simulink model "tank_FP"  (R2021b)
settings: Solver=VariableStepAuto  StartTime=0.0  StopTime=30  RelTol=1e-4
undefined symbols (not defined in the file): A, Ak, B, Be, beta, Bh, Bs, C, d, Dh, Discrete, Dm, Ds, Fc, Flp, Hd, Hm_init, Hs_init, Jh, Ke, Kh, Ks, Mm, Ms, noise, Ph, R, Time, tlcAlpha, Ts, xe
libraries: simulink x3, ctrlSharedLib x2, cstblocks x1
settings Model: Creator=buse  LastModifiedBy=buse

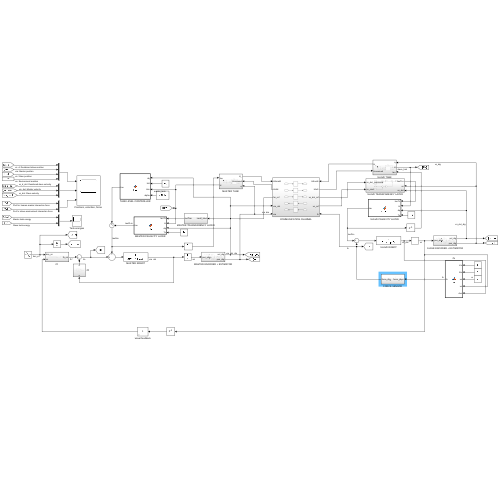
[thumbnail: Simulink's stored preview of the top-level diagram]
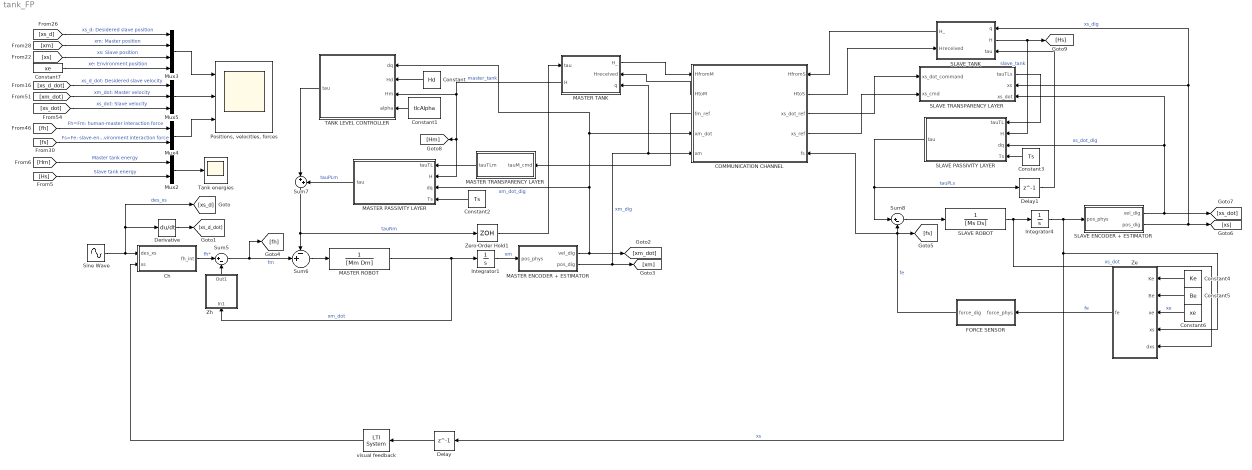
== system tank_FP ==
  COMMUNICATION CHANNEL : Subsystem
      settings: PortSchema="{\"entries\":[{\"content\":{\"sides\":[{\"content\":{\"connectorIds\":[\"In1\",\"Out3\",\"Out4\",\"Out5\",\"In2\"]},\"type\":\"ConnectorPlacement.EquallySpacedRectSide\",\"uuid\":\"1c070cf8-9aa7-4f7b-8e2f-2632c2893f69\"},{\"content\":{\"connectorIds\":[\"In3\",\"Out1\",\"Out2\",\"In4\",\"In5\"],\"side\":\"RIGHT\"},\"type\":\"ConnectorPlacement.EquallySpacedRectSide\",\"uuid\":\"32173565-3523-4dfc-9820-763c87098354\"},{\"content\":{\"connectorIds\":[],\"side\":\"TOP\"},\"type\":\"ConnectorPlacement.EquallySpacedRectSide\",\"uuid\":\"13187df6-bf6f-436e-a2ee-34150977e6a8\"},{\"content\":{\"connectorIds\":[],\"side\":\"HIDDEN\"},\"type\":\"ConnectorPlacement.EquallySpacedRectSide\",\"uuid\":\"1e5bcdd7-6028-40f7-b524-727817e519ff\"}]},\"type\":\"ConnectorPlacement.EquallySpacedConnector\",\"uuid\":\"c84d0440-83b9-4b92-a10a-1f72bb115b54\"}],\"packageUris\":[\"http://schema.mathworks.com/mf0/Connector/R2020b\"],\"version\":\"1.0\"}"
  Ch : Subsystem
  Constant : Constant  Value=Hd
  Constant1 : Constant  Value=tlcAlpha
  Constant2 : Constant  Value=Ts
  Constant3 : Constant  Value=Ts
  Constant4 : Constant  Value=Ke
  Constant5 : Constant  Value=Be
  Constant6 : Constant  Value=xe
  Constant7 : Constant  Value=xe
  Delay : Delay  DelayLength=1  SampleTime=Ts
  Delay1 : Delay  DelayLength=1  SampleTime=Ts
  Derivative : Derivative
  "FORCE SENSOR " : Subsystem
  Integrator1 : Integrator
  Integrator4 : Integrator
  MASTER ENCODER + ESTIMATOR : Subsystem
  MASTER PASSIVITY LAYER : MATLAB Function  TreatAsAtomicUnit=on
  MASTER ROBOT : TransferFcn  Denominator=[Mm Dm]
  MASTER TANK : Subsystem
      settings: PortSchema="{\"entries\":[{\"content\":{\"sides\":[{\"content\":{\"connectorIds\":[\"Out2\",\"In1\",\"In2\"]},\"type\":\"ConnectorPlacement.EquallySpacedRectSide\",\"uuid\":\"482b0a11-f044-49fa-a74d-4dac8b5b787b\"},{\"content\":{\"connectorIds\":[\"In3\",\"Out1\"],\"side\":\"RIGHT\"},\"type\":\"ConnectorPlacement.EquallySpacedRectSide\",\"uuid\":\"b0c369ed-ae40-43d8-b393-bca9f7720d62\"},{\"content\":{\"connectorIds\":[],\"side\":\"TOP\"},\"type\":\"ConnectorPlacement.EquallySpacedRectSide\",\"uuid\":\"ff021616-d6aa-4c0a-874b-a9ebe947c92c\"},{\"content\":{\"connectorIds\":[],\"side\":\"BOTTOM\"},\"type\":\"ConnectorPlacement.EquallySpacedRectSide\",\"uuid\":\"4e18ee96-bca7-41b6-9abb-5b593b41c296\"},{\"content\":{\"connectorIds\":[],\"side\":\"HIDDEN\"},\"type\":\"ConnectorPlacement.EquallySpacedRectSide\",\"uuid\":\"be815b34-35c7-4c6f-8c8b-4a812b3d12e9\"}]},\"type\":\"ConnectorPlacement.EquallySpacedConnector\",\"uuid\":\"78552b8a-5f1c-4815-a807-de98f58b7f2e\"}],\"packageUris\":[\"http://schema.mathworks.com/mf0/Connector/R2020b\"],\"version\":\"1.0\"}"
  MASTER TRANSPARENCY LAYER : Subsystem
  Mux2 : Mux  Inputs=2
  Mux3 : Mux
  Mux4 : Mux  Inputs=2
  Mux5 : Mux  Inputs=3
  "Positions, velocities, forces" : Scope  NumInputPorts=3
  SLAVE ENCODER + ESTIMATOR : Subsystem
  SLAVE PASSIVITY LAYER : MATLAB Function  TreatAsAtomicUnit=on
  SLAVE ROBOT : TransferFcn  Denominator=[Ms Ds]
  SLAVE TANK : Subsystem
      settings: PortSchema="{\"entries\":[{\"content\":{\"sides\":[{\"content\":{\"connectorIds\":[\"In1\",\"Out2\",\"In2\"]},\"type\":\"ConnectorPlacement.EquallySpacedRectSide\",\"uuid\":\"482b0a11-f044-49fa-a74d-4dac8b5b787b\"},{\"content\":{\"connectorIds\":[\"Out1\",\"In3\"],\"side\":\"RIGHT\"},\"type\":\"ConnectorPlacement.EquallySpacedRectSide\",\"uuid\":\"b0c369ed-ae40-43d8-b393-bca9f7720d62\"},{\"content\":{\"connectorIds\":[],\"side\":\"TOP\"},\"type\":\"ConnectorPlacement.EquallySpacedRectSide\",\"uuid\":\"ff021616-d6aa-4c0a-874b-a9ebe947c92c\"},{\"content\":{\"connectorIds\":[],\"side\":\"BOTTOM\"},\"type\":\"ConnectorPlacement.EquallySpacedRectSide\",\"uuid\":\"4e18ee96-bca7-41b6-9abb-5b593b41c296\"},{\"content\":{\"connectorIds\":[],\"side\":\"HIDDEN\"},\"type\":\"ConnectorPlacement.EquallySpacedRectSide\",\"uuid\":\"be815b34-35c7-4c6f-8c8b-4a812b3d12e9\"}]},\"type\":\"ConnectorPlacement.EquallySpacedConnector\",\"uuid\":\"78552b8a-5f1c-4815-a807-de98f58b7f2e\"}],\"packageUris\":[\"http://schema.mathworks.com/mf0/Connector/R2020b\"],\"version\":\"1.0\"}"
  SLAVE TRANSPARENCY LAYER : Subsystem
      settings: PortSchema="{\"entries\":[{\"content\":{\"sides\":[{\"content\":{\"connectorIds\":[\"In1\",\"In2\"]},\"type\":\"ConnectorPlacement.EquallySpacedRectSide\",\"uuid\":\"c8f256d1-8287-4bc6-9264-40c0684f6acd\"},{\"content\":{\"connectorIds\":[\"Out1\",\"In3\",\"In4\"],\"side\":\"RIGHT\"},\"type\":\"ConnectorPlacement.EquallySpacedRectSide\",\"uuid\":\"cb9f571e-93fc-426e-a4f2-aa96ae3bd6b3\"},{\"content\":{\"connectorIds\":[],\"side\":\"TOP\"},\"type\":\"ConnectorPlacement.EquallySpacedRectSide\",\"uuid\":\"b9b91304-f20e-4a66-aa64-b99c686ee85a\"},{\"content\":{\"connectorIds\":[],\"side\":\"HIDDEN\"},\"type\":\"ConnectorPlacement.EquallySpacedRectSide\",\"uuid\":\"c3abcf5a-e3b9-4b9a-a4b1-68c5725be1f4\"}]},\"type\":\"ConnectorPlacement.EquallySpacedConnector\",\"uuid\":\"83907002-acbd-4948-aeba-a43201e13c19\"}],\"packageUris\":[\"http://schema.mathworks.com/mf0/Connector/R2020b\"],\"version\":\"1.0\"}"
  Sine Wave : Sin  Amplitude=A  Frequency=Fc  SampleTime=0
  Sum5 : Sum  Inputs=|+-
  Sum6 : Sum  Inputs=-+|
  Sum7 : Sum  Inputs=|++
  Sum8 : Sum  Inputs=|+-
  TANK LEVEL CONTROLLER : MATLAB Function  TreatAsAtomicUnit=on
  Tank energies : Scope
  Ze : MATLAB Function  TreatAsAtomicUnit=on
  Zero-Order Hold1 : ZeroOrderHold  SampleTime=Ts
  Zh : Subsystem
  visual feedback : cstblocks/LTI System  sys=1  IC=[]
  wires:
  [xs_dot] -> Mux5/3  "xs_dot: Slave velocity"
  Mux5/1 -> "Positions, velocities, forces"/2
  [xs] -> Mux3/3  "xs: Slave position"
  [fh] -> Mux4/1  "Fh=Fm: human-master interaction force"
  Mux4/1 -> "Positions, velocities, forces"/3
  [xm_dot] -> Mux5/2  "xm_dot: Master velocity"
  [xs_d_dot] -> Mux5/1  "xs_d_dot: Desidered slave velocity"
  [xm] -> Mux3/2  "xm: Master position"
  Mux3/1 -> "Positions, velocities, forces"/1
  [fs] -> Mux4/2  "Fs=Fe: slave-environment interaction force"
  Constant7/1 -> Mux3/4  "xe: Environment position"
  [xs_d] -> Mux3/1  "xs_d: Desidered slave position"
  SLAVE ENCODER + ESTIMATOR/2(pos_dig) -> SLAVE TANK/1(q), SLAVE TRANSPARENCY LAYER/3(xs), [xs]  "xs_dig"
  Ze/1(fe) -> "FORCE SENSOR "/1(force_phys)  "fe"
  Constant3/1 -> SLAVE PASSIVITY LAYER/4(Ts)
  Constant6/1 -> Ze/3(xe)  "xe"
  COMMUNICATION CHANNEL/1(HtoM) -> MASTER TANK/1(Hreceived)
  visual feedback/1 -> Ch/2(xs)
  Sum6/1 -> MASTER ROBOT/1
  MASTER PASSIVITY LAYER/1(tau) -> Sum7/2  "tauPLm"
  MASTER TANK/1(H) -> [Hm], MASTER PASSIVITY LAYER/2(H), TANK LEVEL CONTROLLER/3(Hm)  "master_tank"
  MASTER ENCODER + ESTIMATOR/1(vel_dig) -> [xm_dot], TANK LEVEL CONTROLLER/1(dq), COMMUNICATION CHANNEL/4(xm_dot), MASTER PASSIVITY LAYER/3(dq)  "xm_dot_dig"
  MASTER ROBOT/1 -> Zh/1(In1), Integrator1/1  "xm_dot"
  Delay/1 -> visual feedback/1
  MASTER TRANSPARENCY LAYER/1(tauTLm) -> MASTER PASSIVITY LAYER/1(tauTL)
  COMMUNICATION CHANNEL/4(xs_dot_ref) -> SLAVE TRANSPARENCY LAYER/1(xs_dot_command)
  Sum7/1 -> Zero-Order Hold1/1, Sum6/1  "tauRm"
  Integrator1/1 -> MASTER ENCODER + ESTIMATOR/1(pos_phys)  "xm"
  Constant4/1 -> Ze/1(Ke)
  SLAVE ENCODER + ESTIMATOR/1(vel_dig) -> [xs_dot], SLAVE TRANSPARENCY LAYER/4(xs_dot), SLAVE PASSIVITY LAYER/3(dq)  "xs_dot_dig"
  Sum5/1 -> Sum6/2, [fh]  "fm"
  Constant1/1 -> TANK LEVEL CONTROLLER/4(alpha)
  Sine Wave/1 -> Ch/1(des_xs), Derivative/1, [xs_d]  "des_xs"
  Sum8/1 -> SLAVE ROBOT/1
  Zh/1(Out1) -> Sum5/2
  SLAVE TANK/2(H) -> [Hs], SLAVE PASSIVITY LAYER/2(H)  "slave_tank"
  Constant5/1 -> Ze/2(Be)
  COMMUNICATION CHANNEL/2(fm_ref) -> MASTER TRANSPARENCY LAYER/1(tauM_cmd)
  SLAVE PASSIVITY LAYER/1(tau) -> Sum8/1, Delay1/1  "tauPLs"
  Ch/1(fh_int) -> Sum5/1  "fh*"
  SLAVE TANK/1(H_) -> COMMUNICATION CHANNEL/1(HfromS)
  TANK LEVEL CONTROLLER/1(tau) -> Sum7/1
  MASTER TANK/2(H_) -> COMMUNICATION CHANNEL/3(HfromM)
  MASTER ENCODER + ESTIMATOR/2(pos_dig) -> [xm], MASTER TANK/2(q), COMMUNICATION CHANNEL/5(xm)  "xm_dig"
  Constant2/1 -> MASTER PASSIVITY LAYER/4(Ts)
  COMMUNICATION CHANNEL/5(xs_ref) -> SLAVE TRANSPARENCY LAYER/2(xs_cmd)
  Zero-Order Hold1/1 -> MASTER TANK/3(tau)
  Delay1/1 -> SLAVE TANK/2(tau)
  SLAVE TRANSPARENCY LAYER/1(tauTLs) -> SLAVE PASSIVITY LAYER/1(tauTL)
  Constant/1 -> TANK LEVEL CONTROLLER/2(Hd)
  SLAVE ROBOT/1 -> Ze/5(dxs), Integrator4/1  "xs_dot"
  Integrator4/1 -> Delay/1, Ze/4(xs), SLAVE ENCODER + ESTIMATOR/1(pos_phys)  "xs"
  COMMUNICATION CHANNEL/3(HtoS) -> SLAVE TANK/3(Hreceived)
  Derivative/1 -> [xs_d_dot]
  [Hs] -> Mux2/2  "Slave tank energy"
  Mux2/1 -> Tank energies/1
  [Hm] -> Mux2/1  "Master tank energy"
  "FORCE SENSOR "/1(force_dig) -> COMMUNICATION CHANNEL/2(fs), [fs], Sum8/2  "fe"

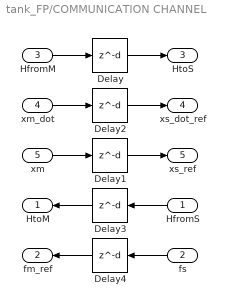
== system tank_FP/COMMUNICATION CHANNEL ==
  HfromS : Inport
  fs : Inport  Port=2
  HfromM : Inport  Port=3
  xm_dot : Inport  Port=4
  xm : Inport  Port=5
  Delay{,1..4} (5 alike) : Delay  DelayLength=d  SampleTime=Ts
  HtoM : Outport
  fm_ref : Outport  Port=2
  HtoS : Outport  Port=3
  xs_dot_ref : Outport  Port=4
  xs_ref : Outport  Port=5
  wires:
  HfromS/1 -> Delay3/1
  xm_dot/1 -> Delay2/1
  fs/1 -> Delay4/1
  Delay4/1 -> fm_ref/1
  xm/1 -> Delay1/1
  Delay1/1 -> xs_ref/1
  Delay2/1 -> xs_dot_ref/1
  HfromM/1 -> Delay/1
  Delay/1 -> HtoS/1
  Delay3/1 -> HtoM/1

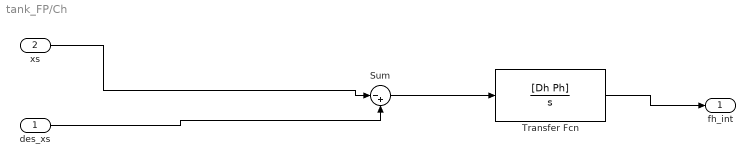
== system tank_FP/Ch ==
  des_xs : Inport
  xs : Inport  Port=2
  Sum : Sum  Inputs=|-+
  Transfer Fcn : TransferFcn  Numerator=[Dh Ph]  Denominator=[1 0]
  fh_int : Outport
  wires:
  xs/1 -> Sum/1
  des_xs/1 -> Sum/2
  Sum/1 -> Transfer Fcn/1
  Transfer Fcn/1 -> fh_int/1

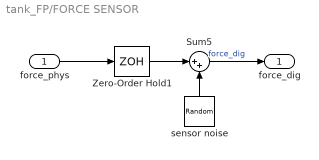
== system tank_FP/FORCE SENSOR  ==
  force_phys : Inport
  Sum5 : Sum  Inputs=|++
  Zero-Order Hold1 : ZeroOrderHold  SampleTime=Ts
  sensor noise : RandomNumber  Variance=0.00000001  SampleTime=Ts
  force_dig : Outport
  wires:
  force_phys/1 -> Zero-Order Hold1/1
  sensor noise/1 -> Sum5/2
  Zero-Order Hold1/1 -> Sum5/1
  Sum5/1 -> force_dig/1  "force_dig"

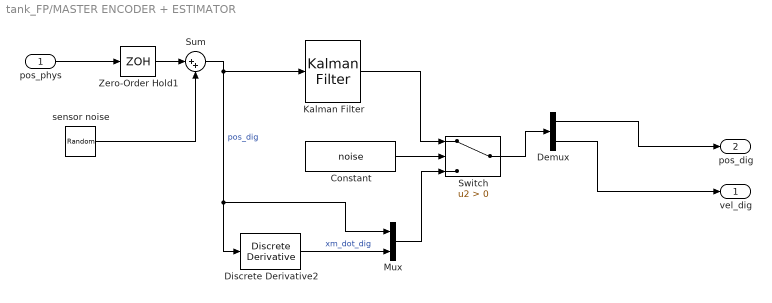
== system tank_FP/MASTER ENCODER + ESTIMATOR ==
  pos_phys : Inport
  Constant : Constant  Value=noise
  Demux : Demux  Outputs=2
  Discrete Derivative2 : simulink/Discrete/Discrete Derivative  gainval=1.0  ICPrevScaledInput=0.0  OutMin=[]  OutMax=[]  OutDataType=fixdt(1, 16)  OutScaling=2^-10  DoSatur=off
  Kalman Filter : ctrlSharedLib/Kalman Filter  TimeDomain=Discrete-Time  UseCurrentEstimator=on  ModelSource=Individual A, B, C, D matrices  ModelSourceVariable=ss(0.95,1,1,0,1)  A=Ak  B=B  C=C  D=0  NumberOfStates=2  NumberOfInputs=1  NumberOfOutputs=1  InitialEstimateSource=Dialog  X0=0  P0=10  UseK=off  UseGH=off  NumberOfProcessNoiseInputs=1  G=1  TimeInvariantG=on  H=0  TimeInvariantH=on  Q=Q_m  TimeInvariantQ=on  R=R  TimeInvariantR=on  N=0  TimeInvariantN=on  AddInputPort=off  AddEnablePort=off  OutputEstimatedY=off  OutputP=off  Ts=Ts
  Mux : Mux  Inputs=2
  Sum : Sum  Inputs=|++
  Switch : Switch  Criteria=u2 > Threshold
  Zero-Order Hold1 : ZeroOrderHold  SampleTime=Ts
  sensor noise : RandomNumber  Variance=noise  SampleTime=Ts
  vel_dig : Outport
  pos_dig : Outport  Port=2
  wires:
  pos_phys/1 -> Zero-Order Hold1/1
  Zero-Order Hold1/1 -> Sum/1
  sensor noise/1 -> Sum/2
  Kalman Filter/1 -> Switch/1
  Sum/1 -> Mux/1, Discrete Derivative2/1, Kalman Filter/1  "pos_dig"
  Constant/1 -> Switch/2
  Mux/1 -> Switch/3
  Discrete Derivative2/1 -> Mux/2  "xm_dot_dig"
  Switch/1 -> Demux/1
  Demux/1 -> pos_dig/1
  Demux/2 -> vel_dig/1

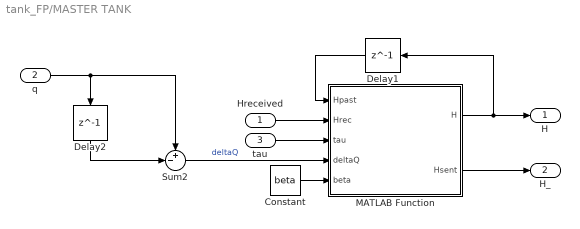
== system tank_FP/MASTER TANK ==
  Hreceived : Inport
  q : Inport  Port=2
  tau : Inport  Port=3
  Constant : Constant  Value=beta
  Delay1 : Delay  DelayLength=1  InitialCondition=Hm_init  SampleTime=Ts
  Delay2 : Delay  DelayLength=1  SampleTime=Ts
  MATLAB Function : MATLAB Function  TreatAsAtomicUnit=on
  Sum2 : Sum  Inputs=+-|
  H : Outport
  H_ : Outport  Port=2
  wires:
  Delay2/1 -> Sum2/2
  q/1 -> Sum2/1, Delay2/1
  MATLAB Function/2(Hsent) -> H_/1
  Constant/1 -> MATLAB Function/5(beta)
  Sum2/1 -> MATLAB Function/4(deltaQ)  "deltaQ"
  Hreceived/1 -> MATLAB Function/2(Hrec)
  tau/1 -> MATLAB Function/3(tau)
  MATLAB Function/1(H) -> Delay1/1, H/1
  Delay1/1 -> MATLAB Function/1(Hpast)

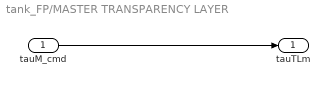
== system tank_FP/MASTER TRANSPARENCY LAYER ==
  tauM_cmd : Inport
  tauTLm : Outport
  wires:
  tauM_cmd/1 -> tauTLm/1

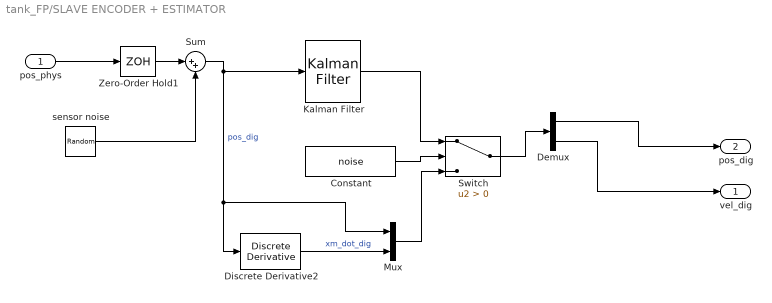
== system tank_FP/SLAVE ENCODER + ESTIMATOR ==
  pos_phys : Inport
  Constant : Constant  Value=noise
  Demux : Demux  Outputs=2
  Discrete Derivative2 : simulink/Discrete/Discrete Derivative  gainval=1.0  ICPrevScaledInput=0.0  OutMin=[]  OutMax=[]  OutDataType=fixdt(1, 16)  OutScaling=2^-10  DoSatur=off
  Kalman Filter : ctrlSharedLib/Kalman Filter  TimeDomain=Discrete-Time  UseCurrentEstimator=on  ModelSource=Individual A, B, C, D matrices  ModelSourceVariable=ss(0.95,1,1,0,1)  A=Ak  B=B  C=C  D=0  NumberOfStates=2  NumberOfInputs=1  NumberOfOutputs=1  InitialEstimateSource=Dialog  X0=0  P0=10  UseK=off  UseGH=off  NumberOfProcessNoiseInputs=1  G=1  TimeInvariantG=on  H=0  TimeInvariantH=on  Q=Q_m  TimeInvariantQ=on  R=R  TimeInvariantR=on  N=0  TimeInvariantN=on  AddInputPort=off  AddEnablePort=off  OutputEstimatedY=off  OutputP=off  Ts=Ts
  Mux : Mux  Inputs=2
  Sum : Sum  Inputs=|++
  Switch : Switch  Criteria=u2 > Threshold
  Zero-Order Hold1 : ZeroOrderHold  SampleTime=Ts
  sensor noise : RandomNumber  Variance=noise  SampleTime=Ts
  vel_dig : Outport
  pos_dig : Outport  Port=2
  wires:
  pos_phys/1 -> Zero-Order Hold1/1
  Zero-Order Hold1/1 -> Sum/1
  sensor noise/1 -> Sum/2
  Kalman Filter/1 -> Switch/1
  Sum/1 -> Mux/1, Discrete Derivative2/1, Kalman Filter/1  "pos_dig"
  Constant/1 -> Switch/2
  Mux/1 -> Switch/3
  Discrete Derivative2/1 -> Mux/2  "xm_dot_dig"
  Switch/1 -> Demux/1
  Demux/1 -> pos_dig/1
  Demux/2 -> vel_dig/1

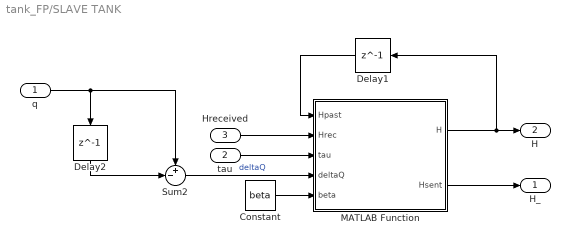
== system tank_FP/SLAVE TANK ==
  q : Inport
  tau : Inport  Port=2
  Hreceived : Inport  Port=3
  Constant : Constant  Value=beta
  Delay1 : Delay  DelayLength=1  InitialCondition=Hs_init  SampleTime=Ts
  Delay2 : Delay  DelayLength=1  SampleTime=Ts
  MATLAB Function : MATLAB Function  TreatAsAtomicUnit=on
  Sum2 : Sum  Inputs=+-|
  H_ : Outport
  H : Outport  Port=2
  wires:
  Delay2/1 -> Sum2/2
  q/1 -> Sum2/1, Delay2/1
  MATLAB Function/2(Hsent) -> H_/1
  Constant/1 -> MATLAB Function/5(beta)
  Sum2/1 -> MATLAB Function/4(deltaQ)  "deltaQ"
  Hreceived/1 -> MATLAB Function/2(Hrec)
  tau/1 -> MATLAB Function/3(tau)
  MATLAB Function/1(H) -> Delay1/1, H/1
  Delay1/1 -> MATLAB Function/1(Hpast)

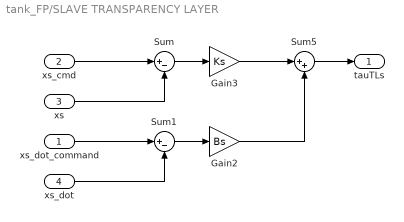
== system tank_FP/SLAVE TRANSPARENCY LAYER ==
  xs_dot_command : Inport
  xs_cmd : Inport  Port=2
  xs : Inport  Port=3
  xs_dot : Inport  Port=4
  Gain2 : Gain  Gain=Bs
  Gain3 : Gain  Gain=Ks
  Sum : Sum  Inputs=|+-
  Sum1 : Sum  Inputs=|+-
  Sum5 : Sum  Inputs=|++
  tauTLs : Outport
  wires:
  Sum5/1 -> tauTLs/1
  xs/1 -> Sum/2
  xs_dot/1 -> Sum1/2
  xs_cmd/1 -> Sum/1
  xs_dot_command/1 -> Sum1/1
  Sum/1 -> Gain3/1
  Sum1/1 -> Gain2/1
  Gain3/1 -> Sum5/1
  Gain2/1 -> Sum5/2

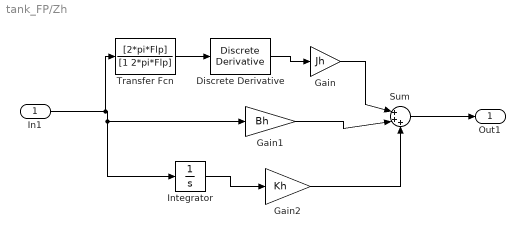
== system tank_FP/Zh ==
  In1 : Inport
  Discrete Derivative : simulink/Discrete/Discrete Derivative  gainval=1.0  ICPrevScaledInput=0.0  OutMin=[]  OutMax=[]  OutDataType=fixdt(1, 16)  OutScaling=2^-10  DoSatur=off
  Gain : Gain  Gain=Jh
  Gain1 : Gain  Gain=Bh
  Gain2 : Gain  Gain=Kh
  Integrator : Integrator
  Sum : Sum  Inputs=|+++
  Transfer Fcn : TransferFcn  Numerator=[2*pi*Flp]  Denominator=[1 2*pi*Flp]
  Out1 : Outport
  wires:
  Discrete Derivative/1 -> Gain/1
  Integrator/1 -> Gain2/1
  In1/1 -> Transfer Fcn/1, Integrator/1, Gain1/1
  Gain/1 -> Sum/1
  Gain1/1 -> Sum/2
  Gain2/1 -> Sum/3
  Sum/1 -> Out1/1
  Transfer Fcn/1 -> Discrete Derivative/1

== matlab function tank_FP/TANK LEVEL CONTROLLER ==
  data: dq input; tau output; Hd input; Hm input; alpha input
function tau = TLC(dq, Hd, Hm, alpha)
% Slide 16
if Hd <= Hm
    d = 0;
else
    d = alpha*(Hd-Hm);
end
tau = -d*dq;

== matlab function tank_FP/MASTER TANK/MATLAB Function ==
  data: Hpast input; H output; Hrec input; tau input; deltaQ input; beta input; Hsent output
function [H,Hsent] = tank(Hpast, Hrec, tau, deltaQ, beta)
Hused = tau*deltaQ;
H = Hpast+Hrec-Hused;    
Hsent = H*beta;
H = H-Hsent; % H k+1

== matlab function tank_FP/SLAVE TANK/MATLAB Function ==
  data: Hpast input; H output; Hrec input; tau input; deltaQ input; beta input; Hsent output
function [H,Hsent] = tank(Hpast, Hrec, tau, deltaQ, beta)
Hused = tau*deltaQ;
H = Hpast+Hrec-Hused;    
Hsent = H*beta;
H = H-Hsent; % H k+1

== matlab function tank_FP/SLAVE PASSIVITY LAYER ==
  data: tauTL input; H input; tau output; dq input; Ts input
function tau = tauPL(tauTL, H, dq,Ts)
% Slide 19
if H<= 0
    tauMax1 = 0;
else
    tauMax1 = tauTL;
end
tauMax2 = H/(dq*Ts);
% Saturated control torque
tau = sign(tauTL)*min([abs(tauMax1),abs(tauMax2)]);

== matlab function tank_FP/MASTER PASSIVITY LAYER ==
  data: tauTL input; H input; tau output; dq input; Ts input
function tau = PL(tauTL, H, dq,Ts)
% Slide 19
if H<= 0
    tauMax1 = 0;
else
    tauMax1 = tauTL;
end
tauMax2 = H/(dq*Ts);
% Saturated control torque
tau = sign(tauTL)*min([abs(tauMax1),abs(tauMax2)]);

== matlab function tank_FP/Ze ==
  data: Ke input; fe output; Be input; xe input; xs input; dxs input
function fe = env(Ke, Be, xe, xs, dxs)
    if xs > xe
        fe = Ke*(xs-xe)+Be*max(dxs, 0);
    else
        fe = 0;
    end
